simulink model "ASMod_TempCatMod"  (R2016b)
settings: configuration reference "CodeGenConfigSet" (kept outside this file)
values from neighbouring files (symbols this model uses):
  ASMod_dvolPFltEG_C = Calibration.Parameter    [init_ASMod_TempCatMod.m]
  PFltLd_resFlw_C = Calibration.Parameter    [init_ASMod_TempCatMod.m]
settings Model: Creator=lenovo  LastModifiedBy=lenovo
settings ConfigSetRef: SourceLocation=Base Workspace

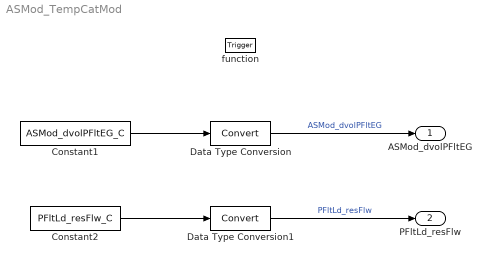
== system ASMod_TempCatMod ==
  function : TriggerPort  TriggerType=function-call  VariantControl=Variant
  Constant1 : Constant  Value=ASMod_dvolPFltEG_C
  Constant2 : Constant  Value=PFltLd_resFlw_C
  Data Type Conversion : DataTypeConversion
  Data Type Conversion1 : DataTypeConversion
  ASMod_dvolPFltEG : Outport  Tag=m^3/h  Description=Calculated exhaust-gas volume flow in the particulate filter  OutMin=0  OutMax=100  OutDataTypeStr=AirVol_m3_h
  PFltLd_resFlw : Outport  Tag=kPa/(m^3/h)  Description=Flow resistance of the particulate filter  Port=2  OutMin=-0.3  OutMax=0.3  OutDataTypeStr=FlowRes_kPa_m3_h
  wires:
  Data Type Conversion/1 -> ASMod_dvolPFltEG/1  "ASMod_dvolPFltEG"
  Data Type Conversion1/1 -> PFltLd_resFlw/1  "PFltLd_resFlw"
  Constant1/1 -> Data Type Conversion/1
  Constant2/1 -> Data Type Conversion1/1
